simulink model "disco_f429_RTOS_blinky"  (R2015a)
settings: Solver=FixedStepDiscrete  SolverMode=SingleTasking  StartTime=0.0  StopTime=10.0  FixedStep=1e-3  RelTol=1e-3
libraries: mbed_targets_stm_disco_f429 x2, simulink x1, mbed_lib x1
settings Model: MbedPath=E:\GitSynology\mbed_target\targets\NUCLEO_F303RE  CovSFcnEnable=off  Creator=oh  LastModifiedBy=oh
settings OptimizationCC: OptimizeModelRefInitCode=on  LifeSpan=1
settings DebuggingCC: SolverPrmCheckMsg=warning
settings HardwareCC: ProdLargestAtomicInteger=Long  ProdLargestAtomicFloat=Double  ProdEndianess=LittleEndian  ProdHWDeviceType=ARM Compatible->ARM Cortex
settings RTWCC: SystemTargetFile=mbed.tlc  TemplateMakefile=mbed.tmf  Description=Mbed Target (Embedded Target)  TargetLang=C++
settings CodeAppCC: IgnoreCustomStorageClasses=off
settings STFCustomTargetCC: CombineOutputUpdateFcns=on  SupportContinuousTime=off  SupportVariableSizeSignals=off  SystemTargetFile=mbed.tlc
settings ERTTargetCC: SupportContinuousTime=off  SupportVariableSizeSignals=off  ERTCustomFileTemplate=mbed_file_process.tlc

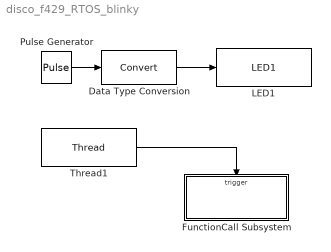
== system disco_f429_RTOS_blinky ==
  Data Type Conversion : DataTypeConversion
  FunctionCall Subsystem : Subsystem  TreatAsAtomicUnit=on
  LED1 : mbed_targets_stm_disco_f429/LED1  Parameter1=0
  Pulse Generator : DiscretePulseGenerator  PulseType=Time based  Period=1  PulseWidth=50
  Thread1 : mbed_lib/RTOS/Thread  ThreadPriority=Normal  SyncFlag=on  Timing=1000  StackOption=Default  StackSize=0
  wires:
  Pulse Generator/1 -> Data Type Conversion/1
  Data Type Conversion/1 -> LED1/1
  Thread1/1 -> FunctionCall Subsystem/Trigger

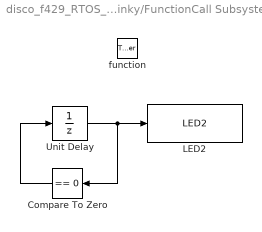
== system disco_f429_RTOS_blinky/FunctionCall Subsystem ==
  function : TriggerPort  TriggerType=function-call
  Compare To Zero : simulink/Logic and Bit Operations/Compare To Zero  relop===  OutDataTypeStr=uint8
  LED2 : mbed_targets_stm_disco_f429/LED2  Parameter1=0
  Unit Delay : UnitDelay  SampleTime=-1
  wires:
  Unit Delay/1 -> LED2/1, Compare To Zero/1
  Compare To Zero/1 -> Unit Delay/1
